simulink model "quad_animation"  (R2017a)
settings: Solver=ode45  StartTime=0.0  StopTime=inf  RelTol=1e-3  EnableMultiTasking=on
undefined symbols (not defined in the file or in its folder): drawPlanarQuad
libraries: simulink x6
settings Model: Creator=ecestudent  LastModifiedBy=jesse
settings DataIOCC: LimitDataPoints=on  SaveFormat=Array
settings OptimizationCC: LifeSpan=inf
settings DebuggingCC: SFUnexpectedBacktrackingDiag=warning  SFNoUnconditionalDefaultTransitionDiag=warning  SFExecutionAtInitializationDiag=none
settings HardwareCC: ProdBitPerPointer=32  ProdBitPerSizeT=32  ProdBitPerPtrDiffT=32  ProdLargestAtomicFloat=None  ProdIntDivRoundTo=Undefined  ProdEndianess=Unspecified  ProdWordSize=32  ProdHWDeviceType=32-bit Generic
settings ModelReferenceCC: PropagateSignalLabelsOutOfModel=off
settings GRTTargetCC: TargetLangStandard=C89/C90 (ANSI)  GeneratePreprocessorConditionals=Disable all
settings ConfigComp: CovMetricSettings=dw  CovHtmlReporting=on  CovSaveCumulativeToWorkspaceVar=on  CovSaveSingleToWorkspaceVar=on  CovExternalEMLEnable=off

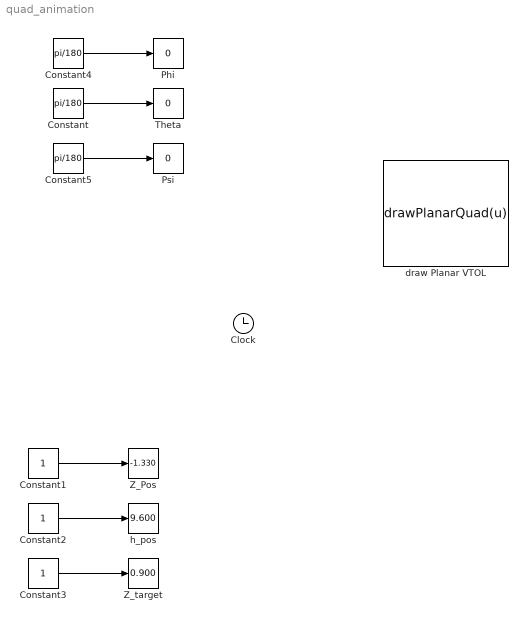
== system quad_animation ==
  Clock : Clock
  Constant : Constant  Value=pi/180
  Constant1 : Constant
  Constant2 : Constant
  Constant3 : Constant
  Constant4 : Constant  Value=pi/180
  Constant5 : Constant  Value=pi/180
  Phi : simulink/Math Operations/Slider Gain  gain=0  low=-60  high=60
  Psi : simulink/Math Operations/Slider Gain  gain=0  low=-180  high=180
  Theta : simulink/Math Operations/Slider Gain  gain=0  low=-60  high=60
  Z_Pos : simulink/Math Operations/Slider Gain  gain=-1.330  low=-3.5  high=3.5
  Z_target : simulink/Math Operations/Slider Gain  gain=0.900  low=-5  high=5
  draw Planar VTOL : MATLABFcn  MATLABFcn=drawPlanarQuad(u)  OutputDimensions=0
      mask Display: image(imread('tv.jpg'))
  h_pos : simulink/Math Operations/Slider Gain  gain=9.600  low=0  high=10
  wires:
  Constant/1 -> Theta/1
  Constant1/1 -> Z_Pos/1
  Constant2/1 -> h_pos/1
  Constant3/1 -> Z_target/1
  Constant4/1 -> Phi/1
  Constant5/1 -> Psi/1
